simulink model "shiftdn35_tb"  (Simulink 7.6)
settings: Solver=ode45  StartTime=0.0  StopTime=1000  RelTol=1e-3
PreLoadFcn:
  | total_errors=0;
undefined symbols (not defined in the file): A, B, xlipgetpartsetting
libraries: xbsIndex_r4 x45, simulink x2, xbsCopyrightNotice_r4 x1
(part 4 of 4)

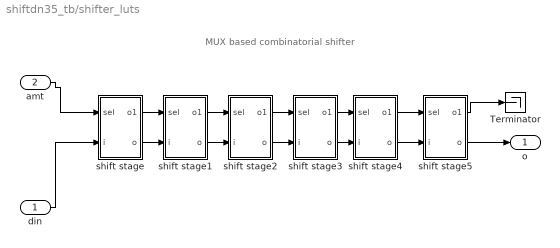
== system shiftdn35_tb/shifter_luts ==
  note: MUX based combinatorial shifter
  din : Inport
  amt : Inport  Port=2
  Terminator : Terminator
  shift stage : Subsystem
  shift stage1 : Subsystem
  shift stage2 : Subsystem
  shift stage3 : Subsystem
  shift stage4 : Subsystem
  shift stage5 : Subsystem
  o : Outport
  wires:
  shift stage/1(o1) -> shift stage1/1(sel)
  shift stage1/1(o1) -> shift stage2/1(sel)
  shift stage2/1(o1) -> shift stage3/1(sel)
  shift stage3/1(o1) -> shift stage4/1(sel)
  shift stage3/2(o) -> shift stage4/2(i)
  shift stage2/2(o) -> shift stage3/2(i)
  shift stage1/2(o) -> shift stage2/2(i)
  shift stage/2(o) -> shift stage1/2(i)
  din/1 -> shift stage/2(i)
  amt/1 -> shift stage/1(sel)
  shift stage5/1(o1) -> Terminator/1
  shift stage4/1(o1) -> shift stage5/1(sel)
  shift stage4/2(o) -> shift stage5/2(i)
  shift stage5/2(o) -> o/1

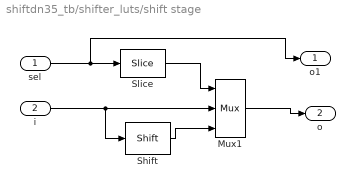
== system shiftdn35_tb/shifter_luts/shift stage ==
  sel : Inport
  i : Inport  Port=2
  Mux1 : xbsIndex_r4/Mux  inputs=2  en=off  latency=0  precision=Full  arith_type="Signed  (2's comp)"  n_bits=8  bin_pt=2  quantization=Truncate  overflow=Wrap  dbl_ovrd=off  block_type=mux
      settings: xl_area=[0, 0, 0, 0, 0, 0, 0]  block_version=VER_STRING_GOES_HERE
  Shift : xbsIndex_r4/Shift  shift_dir=Right  shift_bits=1  en=off  latency=0  precision=Full  arith_type="Signed  (2's comp)"  n_bits=8  bin_pt=2  quantization=Truncate  overflow=Wrap  dbl_ovrd=off  block_type=shift
      settings: xl_area=[0, 0, 0, 0, 0, 0, 0]  block_version=VER_STRING_GOES_HERE
  Slice : xbsIndex_r4/Slice  nbits=1  boolean_output=off  mode=Lower Bit Location + Width  bit1=0  base1=MSB of Input  bit0=0  base0=LSB of Input  dbl_ovrd=off  block_type=slice
      settings: infoedit="Extracts a given range of bits from each input sample and presents it at the output.  The output type is ordinarily unsigned with binary point at zero, but can be Boolean when the slice is one bit wide.<P><P>Hardware notes: In hardware this block costs nothing."  block_version=VER_STRING_GOES_HERE
  o1 : Outport
  o : Outport  Port=2
  wires:
  Slice/1 -> Mux1/1
  Shift/1 -> Mux1/3
  Mux1/1 -> o/1
  i/1 -> Mux1/2, Shift/1
  sel/1 -> o1/1, Slice/1

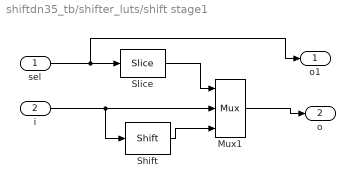
== system shiftdn35_tb/shifter_luts/shift stage1 ==
  sel : Inport
  i : Inport  Port=2
  Mux1 : xbsIndex_r4/Mux  inputs=2  en=off  latency=0  precision=Full  arith_type="Signed  (2's comp)"  n_bits=8  bin_pt=2  quantization=Truncate  overflow=Wrap  dbl_ovrd=off  block_type=mux
      settings: xl_area=[0, 0, 0, 0, 0, 0, 0]  block_version=VER_STRING_GOES_HERE
  Shift : xbsIndex_r4/Shift  shift_dir=Right  shift_bits=2  en=off  latency=0  precision=Full  arith_type="Signed  (2's comp)"  n_bits=8  bin_pt=2  quantization=Truncate  overflow=Wrap  dbl_ovrd=off  block_type=shift
      settings: xl_area=[0, 0, 0, 0, 0, 0, 0]  block_version=VER_STRING_GOES_HERE
  Slice : xbsIndex_r4/Slice  nbits=1  boolean_output=off  mode=Lower Bit Location + Width  bit1=0  base1=MSB of Input  bit0=1  base0=LSB of Input  dbl_ovrd=off  block_type=slice
      settings: infoedit="Extracts a given range of bits from each input sample and presents it at the output.  The output type is ordinarily unsigned with binary point at zero, but can be Boolean when the slice is one bit wide.<P><P>Hardware notes: In hardware this block costs nothing."  block_version=VER_STRING_GOES_HERE
  o1 : Outport
  o : Outport  Port=2
  wires:
  sel/1 -> o1/1, Slice/1
  i/1 -> Shift/1, Mux1/2
  Mux1/1 -> o/1
  Shift/1 -> Mux1/3
  Slice/1 -> Mux1/1

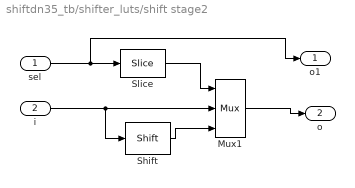
== system shiftdn35_tb/shifter_luts/shift stage2 ==
  sel : Inport
  i : Inport  Port=2
  Mux1 : xbsIndex_r4/Mux  inputs=2  en=off  latency=0  precision=Full  arith_type="Signed  (2's comp)"  n_bits=8  bin_pt=2  quantization=Truncate  overflow=Wrap  dbl_ovrd=off  block_type=mux
      settings: xl_area=[0, 0, 0, 0, 0, 0, 0]  block_version=VER_STRING_GOES_HERE
  Shift : xbsIndex_r4/Shift  shift_dir=Right  shift_bits=4  en=off  latency=0  precision=Full  arith_type="Signed  (2's comp)"  n_bits=8  bin_pt=2  quantization=Truncate  overflow=Wrap  dbl_ovrd=off  block_type=shift
      settings: xl_area=[0, 0, 0, 0, 0, 0, 0]  block_version=VER_STRING_GOES_HERE
  Slice : xbsIndex_r4/Slice  nbits=1  boolean_output=off  mode=Lower Bit Location + Width  bit1=0  base1=MSB of Input  bit0=2  base0=LSB of Input  dbl_ovrd=off  block_type=slice
      settings: infoedit="Extracts a given range of bits from each input sample and presents it at the output.  The output type is ordinarily unsigned with binary point at zero, but can be Boolean when the slice is one bit wide.<P><P>Hardware notes: In hardware this block costs nothing."  block_version=VER_STRING_GOES_HERE
  o1 : Outport
  o : Outport  Port=2
  wires:
  Slice/1 -> Mux1/1
  Shift/1 -> Mux1/3
  Mux1/1 -> o/1
  i/1 -> Mux1/2, Shift/1
  sel/1 -> o1/1, Slice/1

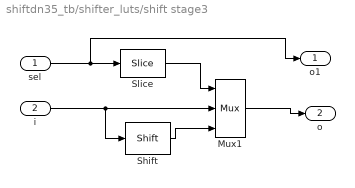
== system shiftdn35_tb/shifter_luts/shift stage3 ==
  sel : Inport
  i : Inport  Port=2
  Mux1 : xbsIndex_r4/Mux  inputs=2  en=off  latency=0  precision=Full  arith_type="Signed  (2's comp)"  n_bits=8  bin_pt=2  quantization=Truncate  overflow=Wrap  dbl_ovrd=off  block_type=mux
      settings: xl_area=[0, 0, 0, 0, 0, 0, 0]  block_version=VER_STRING_GOES_HERE
  Shift : xbsIndex_r4/Shift  shift_dir=Right  shift_bits=8  en=off  latency=0  precision=Full  arith_type="Signed  (2's comp)"  n_bits=8  bin_pt=2  quantization=Truncate  overflow=Wrap  dbl_ovrd=off  block_type=shift
      settings: xl_area=[0, 0, 0, 0, 0, 0, 0]  block_version=VER_STRING_GOES_HERE
  Slice : xbsIndex_r4/Slice  nbits=1  boolean_output=off  mode=Lower Bit Location + Width  bit1=0  base1=MSB of Input  bit0=3  base0=LSB of Input  dbl_ovrd=off  block_type=slice
      settings: infoedit="Extracts a given range of bits from each input sample and presents it at the output.  The output type is ordinarily unsigned with binary point at zero, but can be Boolean when the slice is one bit wide.<P><P>Hardware notes: In hardware this block costs nothing."  block_version=VER_STRING_GOES_HERE
  o1 : Outport
  o : Outport  Port=2
  wires:
  sel/1 -> Slice/1, o1/1
  i/1 -> Shift/1, Mux1/2
  Mux1/1 -> o/1
  Shift/1 -> Mux1/3
  Slice/1 -> Mux1/1

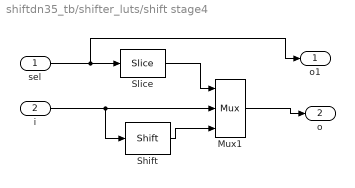
== system shiftdn35_tb/shifter_luts/shift stage4 ==
  sel : Inport
  i : Inport  Port=2
  Mux1 : xbsIndex_r4/Mux  inputs=2  en=off  latency=0  precision=Full  arith_type="Signed  (2's comp)"  n_bits=8  bin_pt=2  quantization=Truncate  overflow=Wrap  dbl_ovrd=off  block_type=mux
      settings: xl_area=[0, 0, 0, 0, 0, 0, 0]  block_version=VER_STRING_GOES_HERE
  Shift : xbsIndex_r4/Shift  shift_dir=Right  shift_bits=16  en=off  latency=0  precision=Full  arith_type="Signed  (2's comp)"  n_bits=8  bin_pt=2  quantization=Truncate  overflow=Wrap  dbl_ovrd=off  block_type=shift
      settings: xl_area=[0, 0, 0, 0, 0, 0, 0]  block_version=VER_STRING_GOES_HERE
  Slice : xbsIndex_r4/Slice  nbits=1  boolean_output=off  mode=Lower Bit Location + Width  bit1=0  base1=MSB of Input  bit0=4  base0=LSB of Input  dbl_ovrd=off  block_type=slice
      settings: infoedit="Extracts a given range of bits from each input sample and presents it at the output.  The output type is ordinarily unsigned with binary point at zero, but can be Boolean when the slice is one bit wide.<P><P>Hardware notes: In hardware this block costs nothing."  block_version=VER_STRING_GOES_HERE
  o1 : Outport
  o : Outport  Port=2
  wires:
  Slice/1 -> Mux1/1
  Shift/1 -> Mux1/3
  Mux1/1 -> o/1
  i/1 -> Mux1/2, Shift/1
  sel/1 -> o1/1, Slice/1

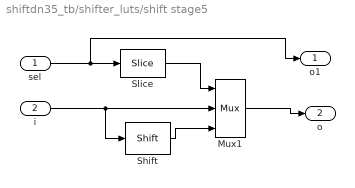
== system shiftdn35_tb/shifter_luts/shift stage5 ==
  sel : Inport
  i : Inport  Port=2
  Mux1 : xbsIndex_r4/Mux  inputs=2  en=off  latency=0  precision=Full  arith_type="Signed  (2's comp)"  n_bits=8  bin_pt=2  quantization=Truncate  overflow=Wrap  dbl_ovrd=off  block_type=mux
      settings: xl_area=[0, 0, 0, 0, 0, 0, 0]  block_version=VER_STRING_GOES_HERE
  Shift : xbsIndex_r4/Shift  shift_dir=Right  shift_bits=32  en=off  latency=0  precision=Full  arith_type="Signed  (2's comp)"  n_bits=8  bin_pt=2  quantization=Truncate  overflow=Wrap  dbl_ovrd=off  block_type=shift
      settings: xl_area=[0, 0, 0, 0, 0, 0, 0]  block_version=VER_STRING_GOES_HERE
  Slice : xbsIndex_r4/Slice  nbits=1  boolean_output=off  mode=Lower Bit Location + Width  bit1=0  base1=MSB of Input  bit0=5  base0=LSB of Input  dbl_ovrd=off  block_type=slice
      settings: infoedit="Extracts a given range of bits from each input sample and presents it at the output.  The output type is ordinarily unsigned with binary point at zero, but can be Boolean when the slice is one bit wide.<P><P>Hardware notes: In hardware this block costs nothing."  block_version=VER_STRING_GOES_HERE
  o1 : Outport
  o : Outport  Port=2
  wires:
  sel/1 -> Slice/1, o1/1
  i/1 -> Shift/1, Mux1/2
  Mux1/1 -> o/1
  Shift/1 -> Mux1/3
  Slice/1 -> Mux1/1
